simulink model "Lab5and6"  (R2024b)
settings: Solver=VariableStepAuto  StartTime=0.0  StopTime=10.0  RelTol=1e-3
libraries: simulink x1
settings Model: Creator=hp  LastModifiedBy=hp

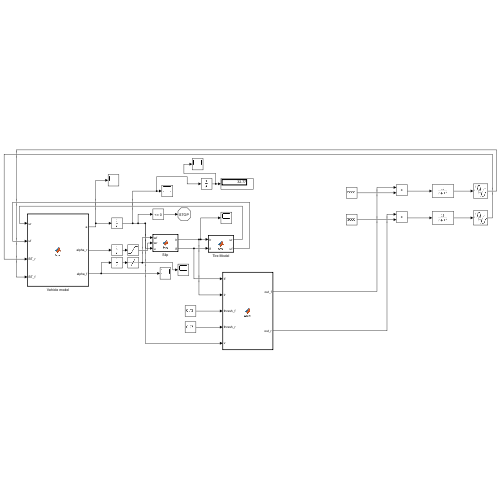
[thumbnail: Simulink's stored preview of the top-level diagram]
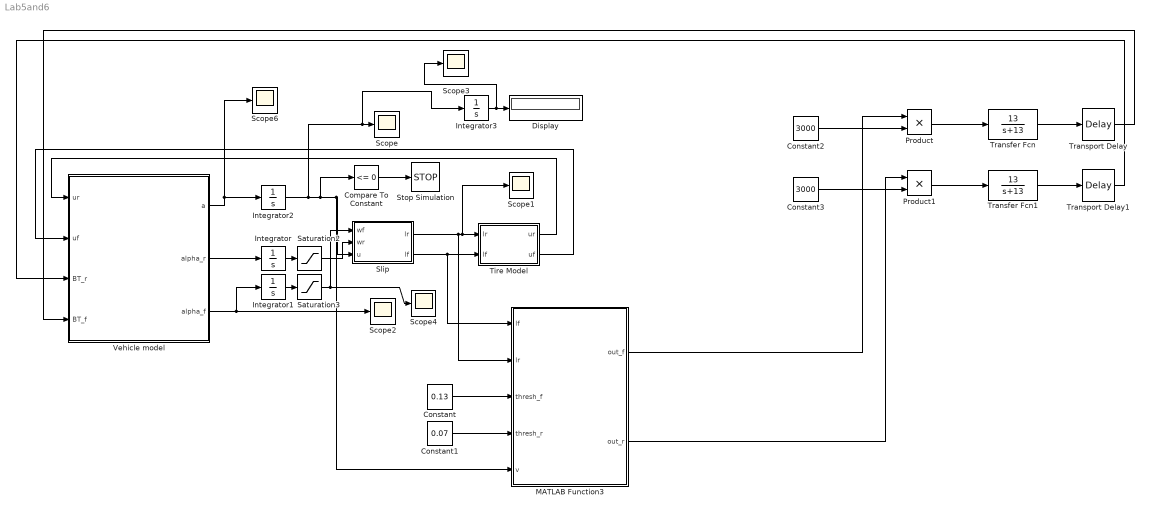
== system Lab5and6 ==
  Compare To Constant : simulink/Logic and Bit Operations/Compare To Constant  relop=<=  const=0  OutDataTypeStr=boolean
  Constant : Constant  Value=0.13
  Constant1 : Constant  Value=0.07
  Constant2 : Constant  Value=3000
  Constant3 : Constant  Value=3000
  Display : Display
  Integrator : Integrator  InitialCondition=37.14
  Integrator1 : Integrator  InitialCondition=37.14
  Integrator2 : Integrator  InitialCondition=13
  Integrator3 : Integrator
  MATLAB Function3 : MATLAB Function  TreatAsAtomicUnit=on
  Product : Product
  Product1 : Product
  Saturation2 : Saturate  UpperLimit=100  LowerLimit=0
  Saturation3 : Saturate  UpperLimit=100  LowerLimit=0
  Scope{,1..4,6} (6 alike) : Scope
  Slip : MATLAB Function  TreatAsAtomicUnit=on
  Stop Simulation : Stop
  Tire Model : MATLAB Function  TreatAsAtomicUnit=on
  Transfer Fcn : TransferFcn  Numerator=[13]  Denominator=[1 13]
  Transfer Fcn1 : TransferFcn  Numerator=[13]  Denominator=[1 13]
  Transport Delay : TransportDelay  DelayTime=0.018
  Transport Delay1 : TransportDelay  DelayTime=0.018
  Vehicle model : MATLAB Function  TreatAsAtomicUnit=on
  wires:
  Slip/1(lr) -> MATLAB Function3/2(lr), Scope1/1, Tire Model/1(lr)
  Slip/2(lf) -> MATLAB Function3/1(lf), Tire Model/2(lf)
  Integrator2/1 -> Integrator3/1, Scope/1, Compare To Constant/1, MATLAB Function3/5(v), Slip/3(u)
  Integrator1/1 -> Saturation3/1
  Compare To Constant/1 -> Stop Simulation/1
  Saturation2/1 -> Slip/2(wr)
  Vehicle model/1(a) -> Scope6/1, Integrator2/1
  Integrator3/1 -> Scope3/1, Display/1
  Tire Model/2(uf) -> Vehicle model/2(uf)
  Saturation3/1 -> Scope4/1, Slip/1(wf)
  Vehicle model/3(alpha_f) -> Integrator1/1, Scope2/1
  Integrator/1 -> Saturation2/1
  Tire Model/1(ur) -> Vehicle model/1(ur)
  Vehicle model/2(alpha_r) -> Integrator/1
  Constant/1 -> MATLAB Function3/3(thresh_f)
  Constant1/1 -> MATLAB Function3/4(thresh_r)
  Product/1 -> Transfer Fcn/1
  Constant2/1 -> Product/2
  Product1/1 -> Transfer Fcn1/1
  Constant3/1 -> Product1/2
  Transfer Fcn/1 -> Transport Delay/1
  Transfer Fcn1/1 -> Transport Delay1/1
  MATLAB Function3/1(out_f) -> Product/1
  MATLAB Function3/2(out_r) -> Product1/1
  Transport Delay/1 -> Vehicle model/4(BT_f)
  Transport Delay1/1 -> Vehicle model/3(BT_r)

== matlab function Lab5and6/Slip ==
  data: wf input; wr input; u input; lr output; lf output
function [lr,lf] = fcn(wf,wr,u)

r=0.35;

if wr*r>u
        wr=u/r;
end

if wf*r>u
        wf=u/r;
end

lf = (u-wf*r) / u;
lr = (u-wr*r) / u;

lf = (-wf * r + u) /(u) ;
lr = (-wr * r + u) /(u) ;

end

== matlab function Lab5and6/Vehicle model ==
  data: a output; ur input; uf input; BT_r input; BT_f input; alpha_r output; alpha_f output
function [a, alpha_r,alpha_f] = fcn(ur,uf,BT_r,BT_f)

W = 2000;
g = 9.8;
L = 3.2;
Lr = 2;
Lf = 1.2;
h = 0.5;
fr = 0.01;
J = 0.7;
r = 0.35;


Wf = (W / L) * (Lr + h * (uf + fr));
Wr = (W / L) * (Lf - h * (ur + fr));

Fbf = uf * Wf;
Fbr = ur * Wr;


a = -(g / W) * (Fbf + Fbr + (fr * W));
alpha_r = -(BT_r - ((Fbr + (fr * Wr)) * r)) / J;
alpha_f = -(BT_f - ((Fbf + (fr * Wf)) * r)) / J;

end

== matlab function Lab5and6/Tire Model ==
  data: lr input; ur output; lf input; uf output
function [ur,uf] = fcn(lr,lf)

ur = sign(lr) * ((0.35) * (1 - exp(-24 * lr)) - (0.1 * lr));
uf = sign(lf) * ((0.35) * (1 - exp(-24 * lf)) - (0.1 * lf));

end

== matlab function Lab5and6/MATLAB Function3 ==
  data: out_f output; out_r output; lf input; lr input; thresh_f input; thresh_r input; v input
function [out_f, out_r] = ABS(lf, lr, thresh_f, thresh_r, v)

    % initialize ABS  status (1 = ABS inactive, 0 = ABS active)
    out_f = 1;
    out_r = 1;

    if lf > thresh_f 
        out_f = 0;
    end

    if lr > thresh_r
        out_r = 0;
    end

    if v < 4
        out_f = 1;
        out_r = 1;
    end

end
